simulink model "linear_simulation_tracking"  (R2023a)
settings: Solver=VariableStepAuto  StartTime=0.0  StopTime=10  RelTol=1e-3
undefined symbols (not defined in the file): A_front, A_side, b_front, b_side, c, init_cond, Ts
libraries: simulink x2
settings Model: Creator=ninj2  LastModifiedBy=morit
settings OptimizationCC: ReuseModelBlockBuffer=off

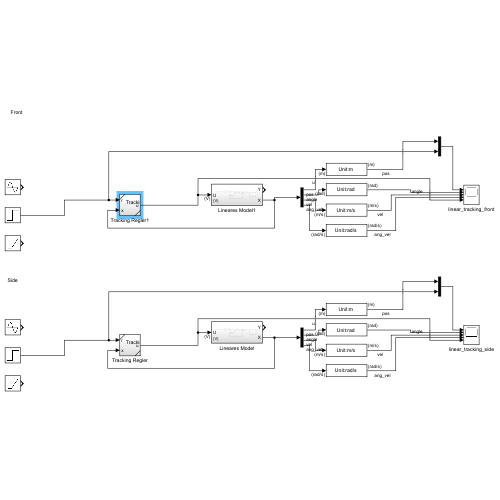
[thumbnail: Simulink's stored preview of the top-level diagram]
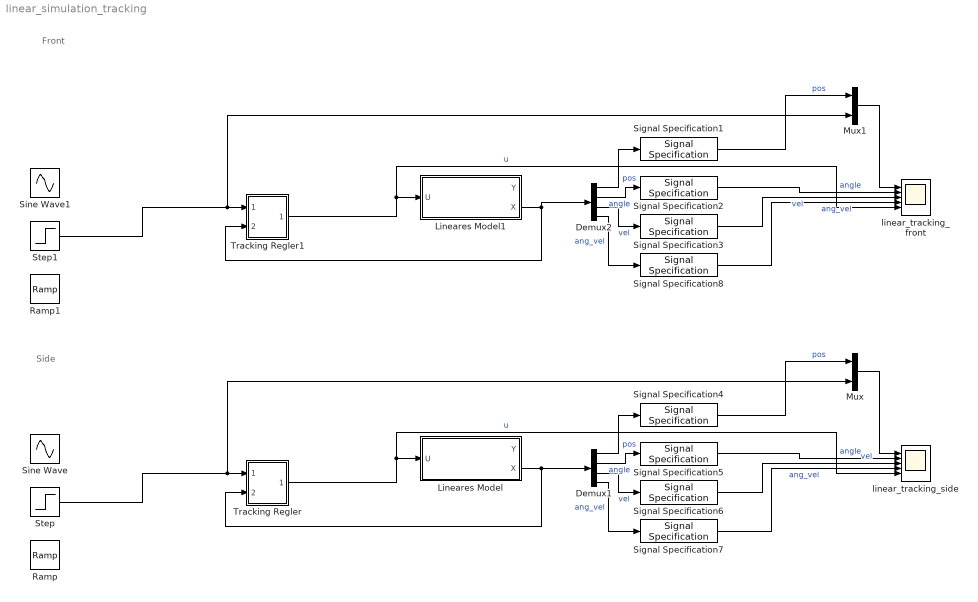
== system linear_simulation_tracking ==
  note: Side
  note: Front
  Demux1 : Demux
  Demux2 : Demux
  Lineares Model : Subsystem
  Lineares Model1 : Subsystem
  Mux : Mux  Inputs=2
  Mux1 : Mux  Inputs=2
  Ramp : simulink/Sources/Ramp  slope=0.01  start=0  InitialOutput=0
  Ramp1 : simulink/Sources/Ramp  slope=0.01  start=0  InitialOutput=0
  Signal Specification1 : SignalSpecification  Unit=m
  Signal Specification2 : SignalSpecification  Unit=rad
  Signal Specification3 : SignalSpecification  Unit=m/s
  Signal Specification4 : SignalSpecification  Unit=m
  Signal Specification5 : SignalSpecification  Unit=rad
  Signal Specification6 : SignalSpecification  Unit=m/s
  Signal Specification7 : SignalSpecification  Unit=rad/s
  Signal Specification8 : SignalSpecification  Unit=rad/s
  Sine Wave : Sin  Amplitude=0.05  Frequency=0.3  SampleTime=0
  Sine Wave1 : Sin  Amplitude=0.05  Frequency=0.3  SampleTime=0
  Step : Step  After=0.05  SampleTime=0
  Step1 : Step  After=0.05  SampleTime=0
  Tracking Regler : Subsystem  ReferencedSubsystem=Tracking_Regler_Side
  Tracking Regler1 : Subsystem  ReferencedSubsystem=Tracking_Regler_Front
  linear_tracking_front : Scope  NumInputPorts=5
  linear_tracking_side : Scope  NumInputPorts=5
  wires:
  Demux1/1 -> Signal Specification4/1  "pos"
  Signal Specification7/1 -> linear_tracking_side/4  "ang_vel"
  Signal Specification6/1 -> linear_tracking_side/3  "vel"
  Demux1/3 -> Signal Specification6/1  "vel"
  Signal Specification4/1 -> Mux/1  "pos"
  Demux1/4 -> Signal Specification7/1  "ang_vel"
  Signal Specification5/1 -> linear_tracking_side/2  "angle"
  Lineares Model/2(X) -> Tracking Regler/2, Demux1/1
  Demux1/2 -> Signal Specification5/1  "angle"
  Mux/1 -> linear_tracking_side/1
  Tracking Regler/1 -> linear_tracking_side/5, Lineares Model/1(U)  "u"
  Step/1 -> Mux/2, Tracking Regler/1
  Signal Specification3/1 -> linear_tracking_front/3  "vel"
  Demux2/2 -> Signal Specification2/1  "angle"
  Step1/1 -> Mux1/2, Tracking Regler1/1
  Lineares Model1/2(X) -> Demux2/1, Tracking Regler1/2
  Signal Specification1/1 -> Mux1/1  "pos"
  Demux2/4 -> Signal Specification8/1  "ang_vel"
  Mux1/1 -> linear_tracking_front/1
  Demux2/3 -> Signal Specification3/1  "vel"
  Signal Specification8/1 -> linear_tracking_front/4  "ang_vel"
  Signal Specification2/1 -> linear_tracking_front/2  "angle"
  Demux2/1 -> Signal Specification1/1  "pos"
  Tracking Regler1/1 -> linear_tracking_front/5, Lineares Model1/1(U)  "u"

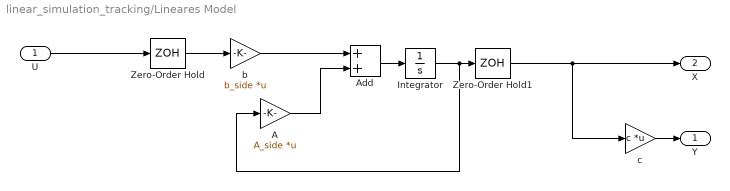
== system linear_simulation_tracking/Lineares Model ==
  U : Inport  Unit=V
  A : Gain  Gain=A_side  Multiplication=Matrix(K*u)
  Add : Sum
  Integrator : Integrator  InitialCondition=init_cond
  Zero-Order Hold : ZeroOrderHold  SampleTime=Ts
  Zero-Order Hold1 : ZeroOrderHold  SampleTime=Ts
  b : Gain  Gain=b_side  Multiplication=Matrix(K*u)
  c : Gain  Gain=c  Multiplication=Matrix(K*u)
  Y : Outport
  X : Outport  Port=2
  wires:
  A/1 -> Add/2
  Add/1 -> Integrator/1
  Integrator/1 -> A/1, Zero-Order Hold1/1
  c/1 -> Y/1
  Zero-Order Hold/1 -> b/1
  b/1 -> Add/1
  Zero-Order Hold1/1 -> c/1, X/1
  U/1 -> Zero-Order Hold/1

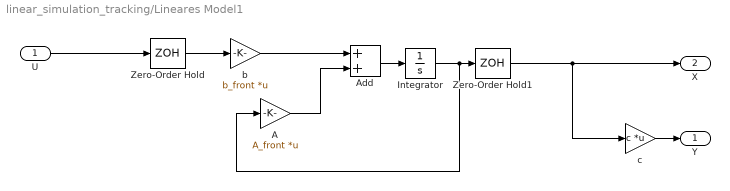
== system linear_simulation_tracking/Lineares Model1 ==
  U : Inport  Unit=V
  A : Gain  Gain=A_front  Multiplication=Matrix(K*u)
  Add : Sum
  Integrator : Integrator  InitialCondition=init_cond
  Zero-Order Hold : ZeroOrderHold  SampleTime=Ts
  Zero-Order Hold1 : ZeroOrderHold  SampleTime=Ts
  b : Gain  Gain=b_front  Multiplication=Matrix(K*u)
  c : Gain  Gain=c  Multiplication=Matrix(K*u)
  Y : Outport
  X : Outport  Port=2
  wires:
  A/1 -> Add/2
  Add/1 -> Integrator/1
  Integrator/1 -> A/1, Zero-Order Hold1/1
  c/1 -> Y/1
  Zero-Order Hold/1 -> b/1
  b/1 -> Add/1
  Zero-Order Hold1/1 -> c/1, X/1
  U/1 -> Zero-Order Hold/1
